simulink model "cic_strukturen0"  (Simulink 7.8)
settings: Solver=ode45  StartTime=0.0  StopTime=10.0  RelTol=1e-3
values from neighbouring files (symbols this model uses):
  M = 2    [CFIR_1.m]    (also in block_lms_.m = 16; cic_dezim1.m = ',num2str(M),'; cic_dezim1_.m = ',num2str(M),     '; cic_dezim2.m = ',num2str(M),')
  R = 4    [CFIR_1.m]    (also in cic_dezim1.m = 10; cic_dezim1_.m = ',num2str(R),'; cic_dezim2.m = 10)
libraries: dspsigops x4
settings Model: Creator=svenhoffmann  LastModifiedBy=josef  ExtModeAutoUpdateStatusClock=off
settings OptimizationCC: InlineInvariantSignals=on  InitFltsAndDblsToZero=on
settings DebuggingCC: SaveWithParameterizedLinksMsg=none  SignalResolutionControl=TryResolveAllWithWarning  MultiTaskDSMMsg=warning  MultiTaskCondExecSysMsg=none  StrictBusMsg=None
settings RTWCC: IncludeERTFirstTime=on
settings GRTTargetCC: TargetFcnLib=ansi_tfl_tmw.mat

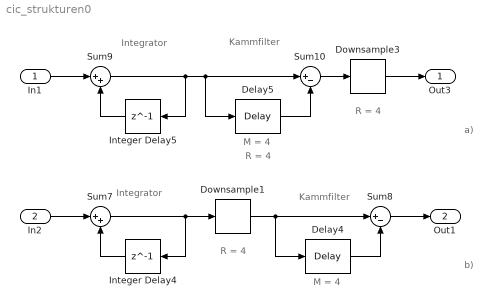
== system cic_strukturen0 ==
  note: M = 4
  note: Integrator
  note: Kammfilter
  note: b)
  note: R = 4
  note: M = 4
  note: Integrator
  note: Kammfilter
  note: a)
  note: R = 4
  note: R = 4
  In1 : Inport
  In2 : Inport  Port=2
  Delay4 : dspsigops/Delay  InputProcessing=Inherited (this choice will be removed - see release notes)  dly_unit=Samples  delay=M  ic_detail=off  dif_ic_for_ch=off  dif_ic_for_dly=off  ic=0  reset_popup=None
  Delay5 : dspsigops/Delay  InputProcessing=Inherited (this choice will be removed - see release notes)  dly_unit=Samples  delay=M*R  ic_detail=off  dif_ic_for_ch=off  dif_ic_for_dly=off  ic=0  reset_popup=None
  Downsample1 : dspsigops/Downsample  N=4  phase=0  InputProcessing=Inherited (this choice will be removed - see release notes)  RateOptions=Enforce single-rate processing  smode=Allow multirate  fmode=Maintain input frame size  ic=0
  Downsample3 : dspsigops/Downsample  N=4  phase=0  InputProcessing=Inherited (this choice will be removed - see release notes)  RateOptions=Enforce single-rate processing  smode=Allow multirate  fmode=Maintain input frame size  ic=0
  Integer Delay4 : Delay  DelayLength=1  InputProcessing=Inherited
  Integer Delay5 : Delay  DelayLength=1  InputProcessing=Inherited
  Sum10 : Sum  Inputs=|+-
  Sum7 : Sum  Inputs=|++
  Sum8 : Sum  Inputs=|+-
  Sum9 : Sum  Inputs=|++
  Out3 : Outport
  Out1 : Outport  Port=2
  wires:
  In2/1 -> Sum7/1
  Sum7/1 -> Integer Delay4/1, Downsample1/1
  Integer Delay4/1 -> Sum7/2
  Delay4/1 -> Sum8/2
  Sum8/1 -> Out1/1
  Downsample1/1 -> Delay4/1, Sum8/1
  In1/1 -> Sum9/1
  Sum9/1 -> Sum10/1, Delay5/1, Integer Delay5/1
  Integer Delay5/1 -> Sum9/2
  Delay5/1 -> Sum10/2
  Sum10/1 -> Downsample3/1
  Downsample3/1 -> Out3/1
